simulink model "test_onoffbutton"  (Simulink 5.0)
settings: Solver=ode5  StartTime=0.0  StopTime=10.0  FixedStep=0.01  RelTol=1e-3
undefined symbols (not defined in the file): sigbuilder_block
CloseFcn:
  | rtwprivate ssgencode ModelCloseRequest test_onoffbutton
settings Model: Creator=riccardo  LastModifiedBy=riccardo  ExtModeMexFile=no_ext_comm  ExtModeAutoUpdateStatusClock=off  RTWSystemTargetFile=ErikaEducational.tlc  RTWTemplateMakefile=ErikaEducational.tmf  RTWGenerateCodeOnly=on  RTWOptions="-aDOWNLCOMM=\"firmdl\" -aDebugLcd=0 -aDownloadToRobot=0 -aERIKABASE=\"/home/riccardo/ErikaEducational/erika\" -aEnforceIntegerDowncast=1 -aFoldNonRolledExpr=1 -aForceParamTrailComments=0 -aGenerateComments=1 -aGenerateReport=0 -aH8RTWLIBDIR=\"/home/riccardo/gencod/lib\" -aIncDataTypeInIds=0 -aIncHierarchyInIds=0 -aInlineInvariantSignals=0 -aInlinedPrmAccess=\"Literals\" -aLEGOTOWERDEVICE=\"/dev/usb/lego0\" -aLocalBlockOutputs=0 -aMaxRTWIdLen=31 -aPrefixModelToSubsysFcnNames=1 -aRTNONFINITE=0 -aRTWVerbose=1 -aRollThreshold=5 -aShowEliminatedStatements=0 -aTaskCF=0 -aUSECUSTCOMM=0 -aUseERT=0 -aVarProcTask=0"

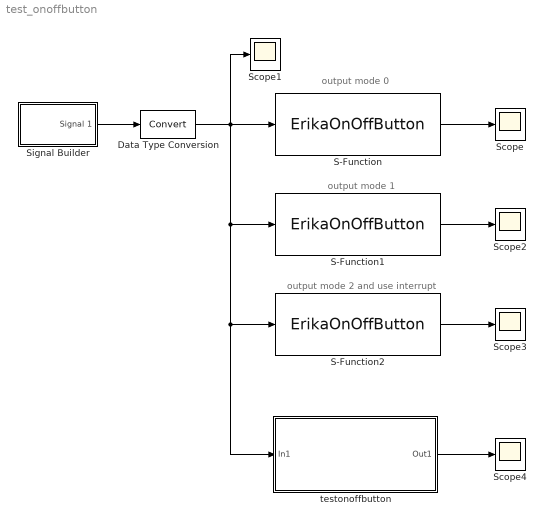
== system test_onoffbutton ==
  note: output mode 0
  note: output mode 1
  note: output mode 2 and use interrupt
  Data Type Conversion : DataTypeConversion  DataType=boolean  SaturateOnIntegerOverflow=on
  S-Function : S-Function  FunctionName=ErikaOnOffButton  Parameters=0 0
  S-Function1 : S-Function  FunctionName=ErikaOnOffButton  Parameters=1 0
  S-Function2 : S-Function  FunctionName=ErikaOnOffButton  Parameters=2 1
  Scope{,1..4} (5 alike) : Scope
      Scope2 settings: SaveName=ScopeData2
      Scope3 settings: SaveName=ScopeData3
      Scope4 settings: SaveName=ScopeData4
  Signal Builder : Subsystem  Tag=STV Subsys  StartFcn=sigbuilder_block('start');  StopFcn=sigbuilder_block('stop');  ClipboardFcn=sigbuilder_block('clipboard');  mask(Sigbuilder block){}
      mask help: Sigbuilder GUI
      mask init:
      | if ~strcmp(get_param(bdroot(gcb),'SimulationStatus'),'stopped') tuvar = sigbuilder_block('maskInit'); end
      settings: CopyFcn=sigbuilder_block('copy');  DeleteFcn=sigbuilder_block('delete');  ModelCloseFcn=sigbuilder_block('modelClose');  PreSaveFcn=sigbuilder_block('preSave');  NameChangeFcn=sigbuilder_block('namechange');  OpenFcn=sigbuilder_block('open',[49.92 52.8 520.32 400.32 ]);  CloseFcn=sigbuilder_block('close');
      mask Display: plot(0,0,100,100,[10,10,40,40,10],[80,20,20,80,80],[40,10],[50,50], [40,27,10],[65,72,56],[40,25,25,10],[28,28,43,43]);
  testonoffbutton : Subsystem
  wires:
  Signal Builder/1(Signal 1) -> Data Type Conversion/1
  S-Function/1 -> Scope/1
  Data Type Conversion/1 -> S-Function/1, Scope1/1, S-Function1/1, S-Function2/1, testonoffbutton/1(In1)
  S-Function1/1 -> Scope2/1
  S-Function2/1 -> Scope3/1
  testonoffbutton/1(Out1) -> Scope4/1

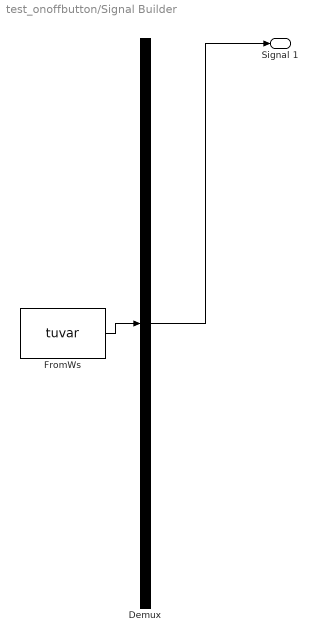
== system test_onoffbutton/Signal Builder ==
  Demux : Demux  Tag=STV Demux  Outputs=1
  FromWs : FromWorkspace  Tag=STV FromWs  VariableName=tuvar  SampleTime=0  SigBuilderData=DataTag0
      SigBuilderData=|
      | channels.label = 'Signal 1'
      | channels.allXData = {[0 4 4 6 6 10]}
      | channels.allYData = {[0 0 1 1 0 0]}
      | dataSet.timeRange = [0 10]
      | dataSet.name = 'Group 1'
  Signal 1 : Outport  Tag=STV Outport
  wires:
  Demux/1 -> Signal 1/1
  FromWs/1 -> Demux/1

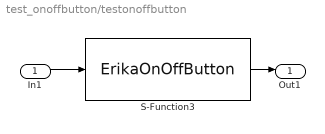
== system test_onoffbutton/testonoffbutton ==
  In1 : Inport
  S-Function3 : S-Function  FunctionName=ErikaOnOffButton  Parameters=1 0
  Out1 : Outport
  wires:
  In1/1 -> S-Function3/1
  S-Function3/1 -> Out1/1
